simulink model "raibert_controller"  (R2018b)
settings: Solver=FixedStepDiscrete  StartTime=0.0  StopTime=inf  FixedStep=sample_time  RelTol=1e-3
InitFcn:
  | addpath('../common/')
  | simulation_params
  | mechanical_params
values from neighbouring files (symbols this model uses):
  sample_time = 1/sample_freq    (= 0.001)    [simulation_params.m]
undefined symbols (not defined in the file or in its folder): F_thrust, Force_Control, K_d_hip, K_p_hip, K_v, sm, v_avg
libraries: powerlib_meascontrol x1
settings Model: Creator=wmartin  LastModifiedBy=akhadke
settings DataIOCC: SaveFormat=StructureWithTime  SaveOutput=off  SignalLogging=off  DSMLogging=off  SaveTime=off
settings OptimizationCC: BlockReduction=off  DefaultParameterBehavior=Inlined  UseFloatMulNetSlope=on  InlineInvariantSignals=on  OptimizeBlockIOStorage=off  BufferReuse=off  GlobalBufferReuse=off  ExpressionFolding=off  LocalBlockOutputs=off  LifeSpan=0.5  SimCompilerOptimization=on  OptimizeDataStoreBuffers=off  BusAssignmentInplaceUpdate=off
settings DebuggingCC: UnderspecifiedInitializationDetection=Classic  MergeDetectMultiDrivingBlocksExec=none  LibraryContextMissingDiagnostic=none
settings HardwareCC: ProdBitPerPointer=32  ProdBitPerSizeT=32  ProdBitPerPtrDiffT=32  ProdLargestAtomicFloat=None  ProdWordSize=32  ProdLongLongMode=on  ProdHWDeviceType=Generic->32-bit x86 compatible
settings ModelReferenceCC: ModelReferenceNumInstancesAllowed=Single  ModelReferenceMinAlgLoopOccurrences=on  PropagateSignalLabelsOutOfModel=off
settings SFSimCC: SimUseLocalCustomCode=off
settings RTWCC: SystemTargetFile=slrt.tlc  TLCOptions=-axPCModelStackSizeKB=1024  TemplateMakefile=slrt_default_tmf  Description=Simulink Real-Time  RTWUseLocalCustomCode=off  CodeExecutionProfiling=on  RTWCompilerOptimization=on
settings CodeAppCC: MaxIdLength=127  StateflowObjectComments=on
settings TargetCC: CodeReplacementLibrary=XPC_BLAS  ParMdlRefBuildCompliant=on  ConcurrentExecutionCompliant=on  GeneratePreprocessorConditionals=Use local settings  MatFileLogging=on  PreserveStateflowLocalDataDimensions=off  MATLABClassNameForMDSCustomization=xpcAperiodicCustomization

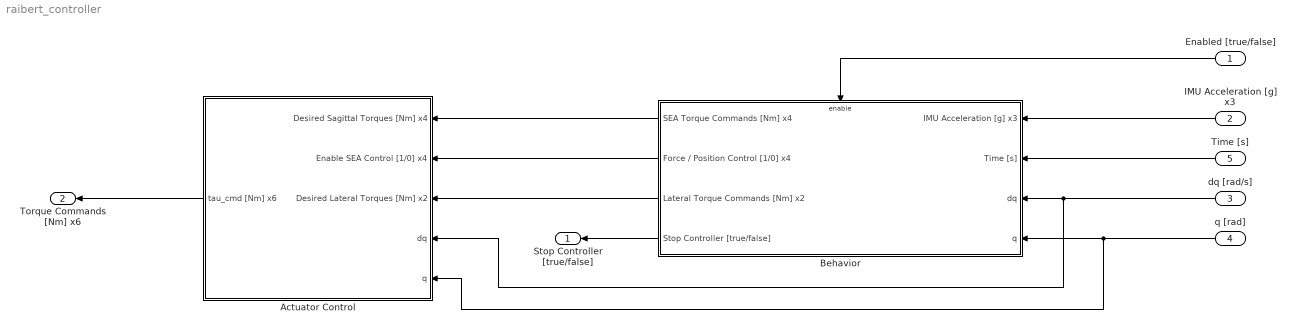
== system raibert_controller ==
  Enabled [true/false] : Inport  OutDataTypeStr=boolean  PortDimensions=1  SampleTime=sample_time  Interpolate=off
  IMU Acceleration [g] x3 : Inport  Port=2  OutDataTypeStr=double  PortDimensions=3  SampleTime=[0.001,0]  Interpolate=off
  dq [rad/s] : Inport  Port=3  OutDataTypeStr=double  PortDimensions=13  SampleTime=[0.001,0]  Interpolate=off
  q [rad] : Inport  Port=4  OutDataTypeStr=double  PortDimensions=13  SampleTime=[0.001,0]  Interpolate=off
  Time [s] : Inport  Port=5  OutDataTypeStr=double  PortDimensions=1  SampleTime=sample_time  Interpolate=off
  Actuator Control : Subsystem
  Behavior : Subsystem
  Stop Controller [true/false] : Outport  OutDataTypeStr=boolean  PortDimensions=1  SampleTime=[0.001,0]  OutputWhenDisabled=reset  InitialOutput=[0 0 0 0 0 0]
  Torque Commands [Nm] x6 : Outport  Port=2  OutDataTypeStr=double  PortDimensions=6  SampleTime=[0.001,0]  OutputWhenDisabled=reset  InitialOutput=[0 0 0 0 0 0]
  wires:
  IMU Acceleration [g] x3/1 -> Behavior/1(IMU Acceleration [g] x3)
  dq [rad/s]/1 -> Behavior/3(dq), Actuator Control/4(dq)
  q [rad]/1 -> Behavior/4(q), Actuator Control/5(q)
  Time [s]/1 -> Behavior/2(Time [s])
  Enabled [true/false]/1 -> Behavior/Enable
  Behavior/4(Stop Controller [true/false]) -> Stop Controller [true/false]/1
  Behavior/2(Force / Position Control [1/0] x4) -> Actuator Control/2(Enable SEA Control [1/0] x4)
  Actuator Control/1(tau_cmd [Nm] x6) -> Torque Commands [Nm] x6/1
  Behavior/1(SEA Torque Commands [Nm] x4) -> Actuator Control/1(Desired Sagittal Torques [Nm] x4)
  Behavior/3(Lateral Torque Commands [Nm] x2) -> Actuator Control/3(Desired Lateral Torques [Nm] x2)

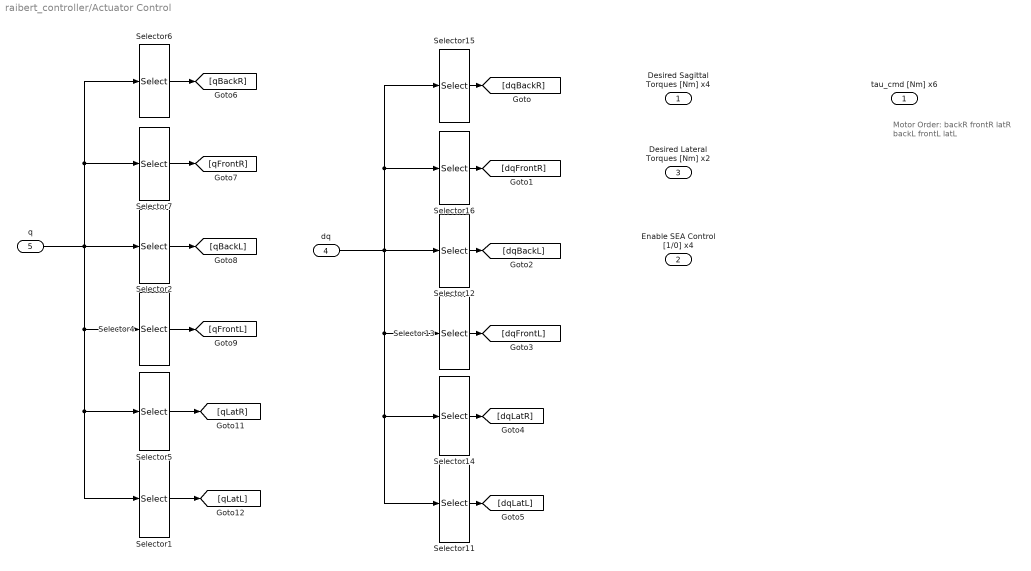
== system raibert_controller/Actuator Control ==
  note: Motor Order:
      |
      | backR
      | frontR
      | latR
      | backL
      | frontL
      | latL
  Desired Sagittal Torques [Nm] x4 : Inport  OutDataTypeStr=double  PortDimensions=4  SampleTime=sample_time
  Enable SEA Control [1/0] x4 : Inport  Port=2  OutDataTypeStr=boolean  PortDimensions=4  SampleTime=sample_time
  Desired Lateral Torques [Nm] x2 : Inport  Port=3  OutDataTypeStr=double  PortDimensions=2  SampleTime=sample_time
  dq : Inport  Port=4  OutDataTypeStr=double  PortDimensions=13  SampleTime=sample_time
  q : Inport  Port=5  OutDataTypeStr=double  PortDimensions=13  SampleTime=sample_time
  Selector1 : Selector  InputPortWidth=13  IndexOptions=Index vector (dialog)  Indices=[10]  OutputSizes=1
  Selector11 : Selector  InputPortWidth=13  IndexOptions=Index vector (dialog)  Indices=[10]  OutputSizes=1
  Selector12 : Selector  InputPortWidth=13  IndexOptions=Index vector (dialog)  Indices=[5 6]  OutputSizes=1
  Selector13 : Selector  InputPortWidth=13  IndexOptions=Index vector (dialog)  Indices=[7 8]  OutputSizes=1
  Selector14 : Selector  InputPortWidth=13  IndexOptions=Index vector (dialog)  Indices=[9]  OutputSizes=1
  Selector15 : Selector  InputPortWidth=13  IndexOptions=Index vector (dialog)  Indices=[1 2]  OutputSizes=1
  Selector16 : Selector  InputPortWidth=13  IndexOptions=Index vector (dialog)  Indices=[3 4]  OutputSizes=1
  Selector2 : Selector  InputPortWidth=13  IndexOptions=Index vector (dialog)  Indices=[5 6]  OutputSizes=1
  Selector4 : Selector  InputPortWidth=13  IndexOptions=Index vector (dialog)  Indices=[7 8]  OutputSizes=1
  Selector5 : Selector  InputPortWidth=13  IndexOptions=Index vector (dialog)  Indices=[9]  OutputSizes=1
  Selector6 : Selector  InputPortWidth=13  IndexOptions=Index vector (dialog)  Indices=[1 2]  OutputSizes=1
  Selector7 : Selector  InputPortWidth=13  IndexOptions=Index vector (dialog)  Indices=[3 4]  OutputSizes=1
  tau_cmd [Nm] x6 : Outport  OutDataTypeStr=double  PortDimensions=6  InitialOutput=[0 0 0 0 0 0]
  wires:
  Selector15/1 -> [dqBackR]
  Selector13/1 -> [dqFrontL]
  Selector1/1 -> [qLatL]
  Selector12/1 -> [dqBackL]
  Selector2/1 -> [qBackL]
  Selector4/1 -> [qFrontL]
  Selector5/1 -> [qLatR]
  Selector6/1 -> [qBackR]
  dq/1 -> Selector12/1, Selector16/1, Selector15/1, Selector13/1, Selector14/1, Selector11/1
  Selector11/1 -> [dqLatL]
  q/1 -> Selector1/1, Selector5/1, Selector4/1, Selector6/1, Selector7/1, Selector2/1
  Selector7/1 -> [qFrontR]
  Selector16/1 -> [dqFrontR]
  Selector14/1 -> [dqLatR]

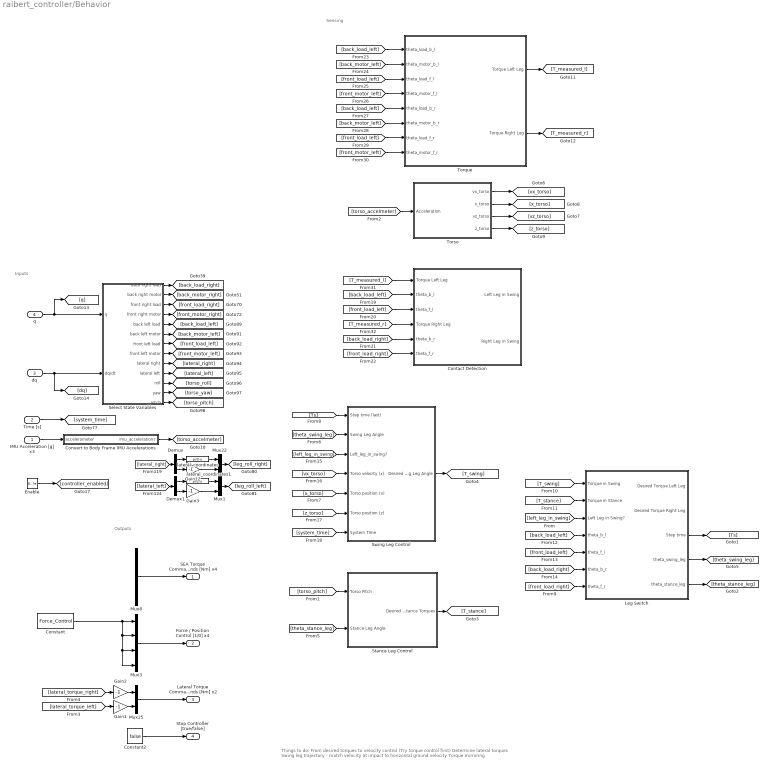
== system raibert_controller/Behavior ==
  note: Things to do:
      | From desired torques to velocity control (Try torque control first)
      | Determine lateral torques
      | Swing leg trajectory - match velocity at impact to horizontal ground velocity
      | Torque mirroring
  note: Outputs
  note: Sensing
  note: Inputs
  IMU Acceleration [g] x3 : Inport  OutDataTypeStr=double  PortDimensions=3  SampleTime=[0.001,0]
  Time [s] : Inport  Port=2  OutDataTypeStr=double  PortDimensions=1  SampleTime=[0.001,0]
  dq : Inport  Port=3  OutDataTypeStr=double  PortDimensions=13  SampleTime=[0.001,0]
  q : Inport  Port=4  OutDataTypeStr=double  PortDimensions=13  SampleTime=[0.001,0]
  Enable : EnablePort  PropagateVarSize=During execution  ShowOutputPort=on
  Constant : Constant  Value=Force_Control
  Constant2 : Constant  Value=false
  Contact Detection : Subsystem
  Convert to Body Frame IMU Accelerations : MATLAB Function  TreatAsAtomicUnit=on
  Demux : Demux  Outputs=2
  Demux1 : Demux  Outputs=2
  Gain{1..3,12} (4 alike) : Gain  Gain=-1
  Leg Switch : Subsystem
  Mux1 : Mux  Inputs=2
  Mux22 : Mux  Inputs=2
  Mux25 : Mux  Inputs=2
  Mux3 : Mux
  Mux8 : Mux
  Select State Variables : Subsystem
  Stance Leg Control : Subsystem  TreatAsAtomicUnit=on
  Swing Leg Control : Subsystem  TreatAsAtomicUnit=on
  Torque : Subsystem
  Torso : Subsystem
  lateral_coordinates : Fcn  Expr=pi/2-u
  lateral_coordinates1 : Fcn  Expr=pi/2-u
  SEA Torque Commands [Nm] x4 : Outport  OutDataTypeStr=double  PortDimensions=4  SampleTime=[0.001,0]  OutputWhenDisabled=reset  InitialOutput=[0 0 0 0]
  Force / Position Control [1/0] x4 : Outport  Port=2  OutDataTypeStr=boolean  PortDimensions=4  SampleTime=[0.001,0]  OutputWhenDisabled=reset  InitialOutput=[0 0 0 0]
  Lateral Torque Commands [Nm] x2 : Outport  Port=3  OutDataTypeStr=double  PortDimensions=2  SampleTime=[0.001,0]  OutputWhenDisabled=reset  InitialOutput=[0 0]
  Stop Controller [true/false] : Outport  Port=4  OutDataTypeStr=boolean  PortDimensions=1  SampleTime=[0.001,0]  OutputWhenDisabled=reset  InitialOutput=0
  wires:
  Time [s]/1 -> [system_time]
  Demux/2 -> Gain12/1
  lateral_coordinates/1 -> Mux22/1
  Gain12/1 -> Mux22/2
  Mux22/1 -> [leg_roll_right]
  Demux/1 -> lateral_coordinates/1
  [lateral_torque_right] -> Gain2/1
  q/1 -> [q], Select State Variables/1(q)
  [lateral_torque_left] -> Gain1/1
  Mux8/1 -> SEA Torque Commands [Nm] x4/1
  Mux3/1 -> Force / Position Control [1/0] x4/1
  Gain2/1 -> Mux25/1
  Mux25/1 -> Lateral Torque Commands [Nm] x2/1
  Gain1/1 -> Mux25/2
  Constant2/1 -> Stop Controller [true/false]/1
  dq/1 -> [dq], Select State Variables/2(dq/dt)
  Select State Variables/1(back right load) -> [back_load_right]
  Select State Variables/2(back right motor) -> [back_motor_right]
  Select State Variables/3(front right load) -> [front_load_right]
  Select State Variables/4(front right motor) -> [front_motor_right]
  Select State Variables/5(back left load) -> [back_load_left]
  Select State Variables/6(back left motor) -> [back_motor_left]
  Select State Variables/7(front left load) -> [front_load_left]
  Select State Variables/8(front left motor) -> [front_motor_left]
  Select State Variables/13(pitch) -> [torso_pitch]
  Select State Variables/12(yaw) -> [torso_yaw]
  Select State Variables/11(roll) -> [torso_roll]
  Select State Variables/10(lateral left) -> [lateral_left]
  Select State Variables/9(lateral right) -> [lateral_right]
  [lateral_right] -> Demux/1
  [lateral_left] -> Demux1/1
  Demux1/1 -> lateral_coordinates1/1
  Mux1/1 -> [leg_roll_left]
  Gain3/1 -> Mux1/2
  lateral_coordinates1/1 -> Mux1/1
  Demux1/2 -> Gain3/1
  Enable/1 -> [controller_enabled]
  Convert to Body Frame IMU Accelerations/1(imu_accelerations) -> [torso_accelmeter]
  IMU Acceleration [g] x3/1 -> Convert to Body Frame IMU Accelerations/1(accelerometer)
  Leg Switch/3(Step time) -> [Ts]
  [torso_pitch] -> Stance Leg Control/1(Torso Pitch)
  [vx_torso] -> Swing Leg Control/4(Torso velocity (x))
  [Ts] -> Swing Leg Control/1(Step time (last))
  [torso_accelmeter] -> Torso/1(Acceleration)
  Stance Leg Control/1(Desired Stance Torques) -> [T_stance]
  Swing Leg Control/1(Desired Swing Leg Angle) -> [T_swing]
  [T_swing] -> Leg Switch/1(Torque in Swing)
  [T_stance] -> Leg Switch/2(Torque in Stance)
  [back_load_right] -> Leg Switch/6(theta_b_r)
  [front_load_right] -> Leg Switch/7(theta_f_r)
  [back_load_left] -> Leg Switch/4(theta_b_l)
  [front_load_left] -> Leg Switch/5(theta_f_l)
  Leg Switch/4(theta_swing_leg) -> [theta_swing_leg]
  [theta_swing_leg] -> Swing Leg Control/2(Swing Leg Angle)
  Constant/1 -> Mux3/4, Mux3/3, Mux3/2, Mux3/1
  [left_leg_in_swing] -> Leg Switch/3("Left Leg in Swing? ")
  [left_leg_in_swing] -> Swing Leg Control/3(Left_leg_in_swing?)
  Torso/1(vx_torso) -> [vx_torso]
  Torso/3(vz_torso) -> [vz_torso]
  Torso/2(x_torso) -> [x_torso]
  Torso/4(z_torso) -> [z_torso]
  [x_torso] -> Swing Leg Control/5(Torso position (x))
  [z_torso] -> Swing Leg Control/6(Torso position (z))
  [system_time] -> Swing Leg Control/7(System Time)
  Leg Switch/5(theta_stance_leg) -> [theta_stance_leg]
  [theta_stance_leg] -> Stance Leg Control/2(Stance Leg Angle)
  [back_load_left] -> Contact Detection/2(theta_b_l)
  [front_load_left] -> Contact Detection/3(theta_f_l)
  [back_load_right] -> Contact Detection/5(theta_b_r)
  [front_load_right] -> Contact Detection/6(theta_f_r)
  [back_load_left] -> Torque/1(theta_load_b_l)
  [back_motor_left] -> Torque/2(theta_motor_b_l)
  [front_load_left] -> Torque/3(theta_load_f_l)
  [front_motor_left] -> Torque/4(theta_motor_f_l)
  [back_load_left] -> Torque/5(theta_load_b_r)
  [back_motor_left] -> Torque/6(theta_motor_b_r)
  [front_load_left] -> Torque/7(theta_load_f_r)
  [front_motor_left] -> Torque/8(theta_motor_f_r)
  Torque/1(Torque Left Leg) -> [T_measured_l]
  Torque/2(Torque Right Leg) -> [T_measured_r]
  [T_measured_l] -> Contact Detection/1(Torque Left Leg)
  [T_measured_r] -> Contact Detection/4(Torque Right Leg)

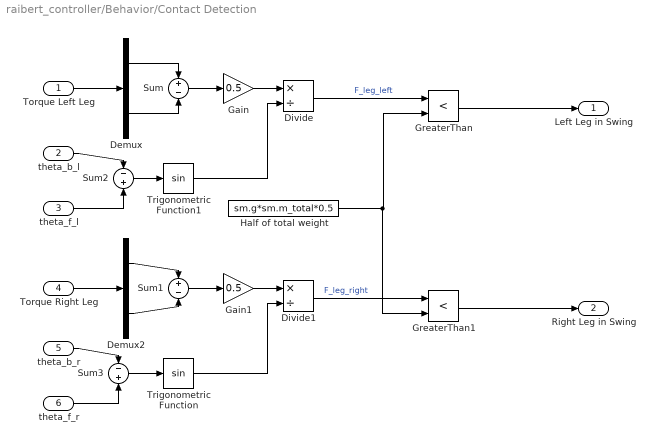
== system raibert_controller/Behavior/Contact Detection ==
  Torque Left Leg : Inport
  theta_b_l : Inport  Port=2
  theta_f_l : Inport  Port=3
  Torque Right Leg : Inport  Port=4
  theta_b_r : Inport  Port=5
  theta_f_r : Inport  Port=6
  Demux : Demux  Outputs=2
  Demux2 : Demux  Outputs=2
  Divide : Product  Inputs=*/
  Divide1 : Product  Inputs=*/
  Gain : Gain  Gain=0.5
  Gain1 : Gain  Gain=0.5
  GreaterThan : RelationalOperator  Operator=<  OutDataTypeStr=boolean  RndMeth=Simplest
  GreaterThan1 : RelationalOperator  Operator=<  OutDataTypeStr=boolean  RndMeth=Simplest
  Half of total weight : Constant  Value=sm.g*sm.m_total*0.5
  Sum : Sum  Inputs=+-
  Sum1 : Sum  Inputs=+-
  Sum2 : Sum  Inputs=-+
  Sum3 : Sum  Inputs=-+
  Trigonometric Function : Trigonometry
  Trigonometric Function1 : Trigonometry
  Left Leg in Swing : Outport
  Right Leg in Swing : Outport  Port=2
  wires:
  Torque Left Leg/1 -> Demux/1
  Demux/1 -> Sum/1
  Demux/2 -> Sum/2
  Torque Right Leg/1 -> Demux2/1
  Demux2/1 -> Sum1/1
  Demux2/2 -> Sum1/2
  Sum/1 -> Gain/1
  Sum1/1 -> Gain1/1
  theta_f_l/1 -> Sum2/2
  theta_b_l/1 -> Sum2/1
  theta_f_r/1 -> Sum3/2
  theta_b_r/1 -> Sum3/1
  Sum3/1 -> Trigonometric Function/1
  Sum2/1 -> Trigonometric Function1/1
  Gain/1 -> Divide/1
  Trigonometric Function1/1 -> Divide/2
  Gain1/1 -> Divide1/1
  Trigonometric Function/1 -> Divide1/2
  Divide/1 -> GreaterThan/1  "F_leg_left"
  Divide1/1 -> GreaterThan1/1  "F_leg_right"
  Half of total weight/1 -> GreaterThan1/2, GreaterThan/2
  GreaterThan/1 -> Left Leg in Swing/1
  GreaterThan1/1 -> Right Leg in Swing/1

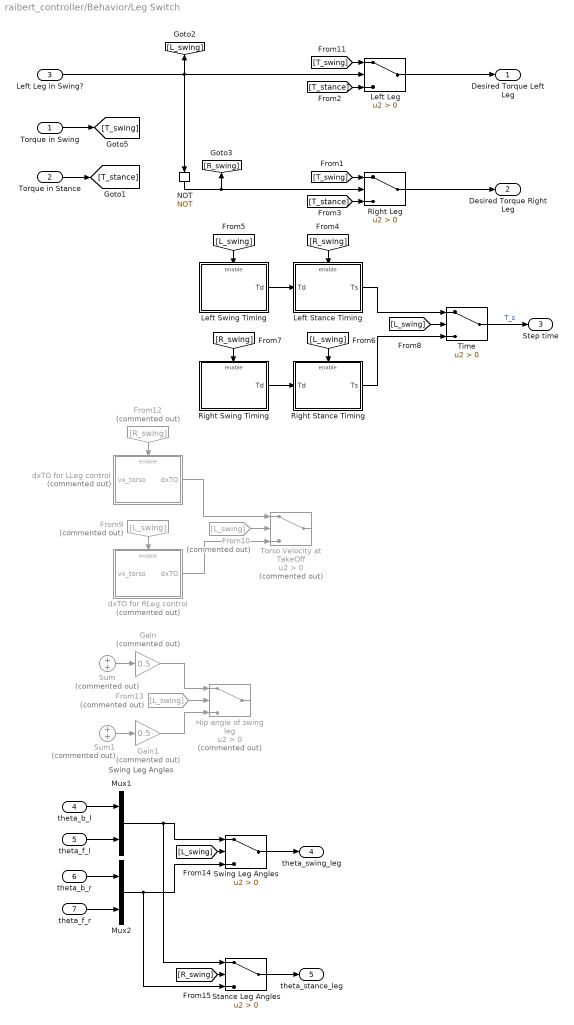
== system raibert_controller/Behavior/Leg Switch ==
  note: Swing Leg Angles
  Torque in Swing : Inport
  Torque in Stance : Inport  Port=2
  "Left Leg in Swing? " : Inport  Port=3
  theta_b_l : Inport  Port=4
  theta_f_l : Inport  Port=5
  theta_b_r : Inport  Port=6
  theta_f_r : Inport  Port=7
  From10 : From  Commented=on  GotoTag=L_swing
  From12 : From  Commented=on  GotoTag=R_swing
  From13 : From  Commented=on  GotoTag=L_swing
  From9 : From  Commented=on  GotoTag=L_swing
  Gain : Gain  Commented=on  Gain=0.5
  Gain1 : Gain  Commented=on  Gain=0.5
  Hip angle of swing leg : Switch  Commented=on  Criteria=u2 > Threshold
  Left Leg : Switch  Criteria=u2 > Threshold
  Left Stance Timing : Subsystem
  Left Swing Timing : Subsystem
  Mux1 : Mux  Inputs=2
  Mux2 : Mux  Inputs=2
  NOT : Logic  Operator=NOT  IconShape=distinctive  AllPortsSameDT=off  OutDataTypeStr=boolean
  Right Leg : Switch  Criteria=u2 > Threshold
  Right Stance Timing : Subsystem
  Right Swing Timing : Subsystem
  Stance Leg Angles : Switch  Criteria=u2 > Threshold
  Sum : Sum  Commented=on
  Sum1 : Sum  Commented=on
  Swing Leg Angles : Switch  Criteria=u2 > Threshold
  Time : Switch  Criteria=u2 > Threshold
  Torso Velocity at TakeOff : Switch  Commented=on  Criteria=u2 > Threshold
  dxTO for LLeg control : Subsystem  Commented=on
  dxTO for RLeg control : Subsystem  Commented=on
  Desired Torque Left Leg : Outport
  Desired Torque Right Leg : Outport  Port=2
  Step time : Outport  Port=3
  theta_swing_leg : Outport  Port=4
  theta_stance_leg : Outport  Port=5
  wires:
  "Left Leg in Swing? "/1 -> NOT/1, Left Leg/2, [L_swing]
  NOT/1 -> [R_swing], Right Leg/2
  Torque in Swing/1 -> [T_swing]
  Torque in Stance/1 -> [T_stance]
  [T_swing] -> Left Leg/1
  [T_swing] -> Right Leg/1
  [T_stance] -> Left Leg/3
  [T_stance] -> Right Leg/3
  Left Leg/1 -> Desired Torque Left Leg/1
  Left Swing Timing/1(Td) -> Left Stance Timing/1(Td)
  Right Swing Timing/1(Td) -> Right Stance Timing/1(Td)
  [L_swing] -> Left Swing Timing/Enable
  [L_swing] -> Right Stance Timing/Enable
  [R_swing] -> Left Stance Timing/Enable
  [R_swing] -> Right Swing Timing/Enable
  Time/1 -> Step time/1  "T_s"
  Left Stance Timing/1(Ts) -> Time/1
  Right Stance Timing/1(Ts) -> Time/3
  [L_swing] -> Time/2
  From9/1 -> dxTO for RLeg control/Enable
  From12/1 -> dxTO for LLeg control/Enable
  dxTO for LLeg control/1(dxTO) -> Torso Velocity at TakeOff/1
  From10/1 -> Torso Velocity at TakeOff/2
  dxTO for RLeg control/1(dxTO) -> Torso Velocity at TakeOff/3
  Sum/1 -> Gain/1
  Sum1/1 -> Gain1/1
  From13/1 -> Hip angle of swing leg/2
  Gain/1 -> Hip angle of swing leg/1
  Gain1/1 -> Hip angle of swing leg/3
  theta_b_l/1 -> Mux1/1
  theta_f_l/1 -> Mux1/2
  theta_b_r/1 -> Mux2/1
  theta_f_r/1 -> Mux2/2
  [L_swing] -> Swing Leg Angles/2
  Swing Leg Angles/1 -> theta_swing_leg/1
  Stance Leg Angles/1 -> theta_stance_leg/1
  Mux2/1 -> Stance Leg Angles/3, Swing Leg Angles/3
  Mux1/1 -> Stance Leg Angles/1, Swing Leg Angles/1
  [R_swing] -> Stance Leg Angles/2
  Right Leg/1 -> Desired Torque Right Leg/1

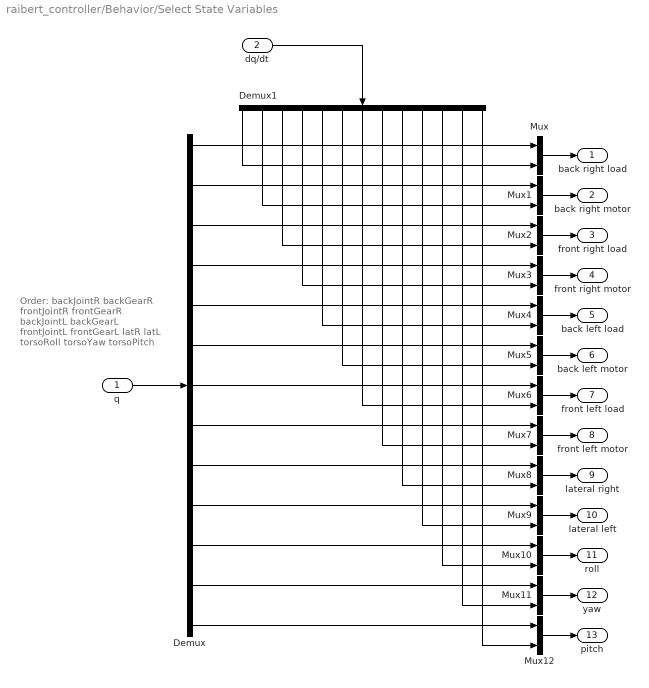
== system raibert_controller/Behavior/Select State Variables ==
  note: Order:
      |
      | backJointR
      | backGearR
      | frontJointR
      | frontGearR
      |
      | backJointL
      | backGearL
      | frontJointL
      | frontGearL
      |
      | latR
      | latL
      |
      | torsoRoll
      | torsoYaw
      | torsoPitch
  q : Inport
  dq/dt : Inport  Port=2
  Demux : Demux  Outputs=13
  Demux1 : Demux  Outputs=13
  Mux{,1..12} (13 alike) : Mux  Inputs=2
  back right load : Outport
  back right motor : Outport  Port=2
  front right load : Outport  Port=3
  front right motor : Outport  Port=4
  back left load : Outport  Port=5
  back left motor : Outport  Port=6
  front left load : Outport  Port=7
  front left motor : Outport  Port=8
  lateral right : Outport  Port=9
  lateral left : Outport  Port=10
  roll : Outport  Port=11
  yaw : Outport  Port=12
  pitch : Outport  Port=13
  wires:
  q/1 -> Demux/1
  dq/dt/1 -> Demux1/1
  Mux/1 -> back right load/1
  Mux1/1 -> back right motor/1
  Mux4/1 -> back left load/1
  Mux5/1 -> back left motor/1
  Mux8/1 -> lateral right/1
  Mux9/1 -> lateral left/1
  Mux12/1 -> pitch/1
  Mux2/1 -> front right load/1
  Mux3/1 -> front right motor/1
  Mux6/1 -> front left load/1
  Mux7/1 -> front left motor/1
  Mux10/1 -> roll/1
  Mux11/1 -> yaw/1
  Demux/1 -> Mux/1
  Demux1/1 -> Mux/2
  Demux/2 -> Mux1/1
  Demux/3 -> Mux2/1
  Demux/4 -> Mux3/1
  Demux/5 -> Mux4/1
  Demux/6 -> Mux5/1
  Demux/7 -> Mux6/1
  Demux/8 -> Mux7/1
  Demux/9 -> Mux8/1
  Demux/10 -> Mux9/1
  Demux/11 -> Mux10/1
  Demux/12 -> Mux11/1
  Demux/13 -> Mux12/1
  Demux1/2 -> Mux1/2
  Demux1/3 -> Mux2/2
  Demux1/4 -> Mux3/2
  Demux1/5 -> Mux4/2
  Demux1/6 -> Mux5/2
  Demux1/7 -> Mux6/2
  Demux1/8 -> Mux7/2
  Demux1/9 -> Mux8/2
  Demux1/10 -> Mux9/2
  Demux1/11 -> Mux10/2
  Demux1/12 -> Mux11/2
  Demux1/13 -> Mux12/2

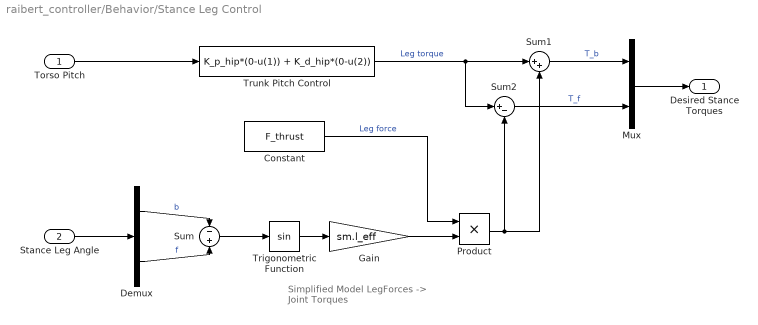
== system raibert_controller/Behavior/Stance Leg Control ==
  note: Simplified Model
      | LegForces -> Joint Torques
  Torso Pitch : Inport
  Stance Leg Angle : Inport  Port=2
  Constant : Constant  Value=F_thrust
  Demux : Demux  Outputs=2
  Gain : Gain  Gain=sm.l_eff
  Mux : Mux  Inputs=2
  Product : Product
  Sum : Sum  Inputs=-+
  Sum1 : Sum  Inputs=|++
  Sum2 : Sum  Inputs=|+-
  Trigonometric Function : Trigonometry
  Trunk Pitch Control : Fcn  Expr=K_p_hip*(0-u(1)) + K_d_hip*(0-u(2))
  Desired Stance Torques : Outport  OutputWhenDisabled=reset  InitialOutput=0
  wires:
  Torso Pitch/1 -> Trunk Pitch Control/1
  Trunk Pitch Control/1 -> Sum2/1, Sum1/1  "Leg torque"
  Mux/1 -> Desired Stance Torques/1
  Constant/1 -> Product/1  "Leg force"
  Stance Leg Angle/1 -> Demux/1
  Demux/1 -> Sum/1  "b"
  Demux/2 -> Sum/2  "f"
  Sum/1 -> Trigonometric Function/1
  Trigonometric Function/1 -> Gain/1
  Gain/1 -> Product/2
  Product/1 -> Sum1/2, Sum2/2
  Sum2/1 -> Mux/2  "T_f"
  Sum1/1 -> Mux/1  "T_b"

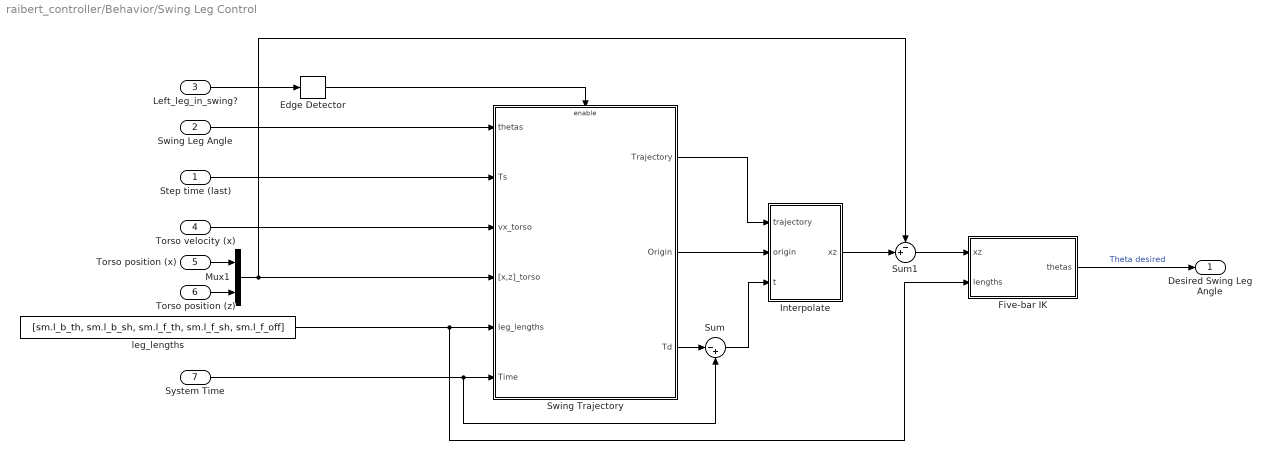
== system raibert_controller/Behavior/Swing Leg Control ==
  Step time (last) : Inport
  Swing Leg Angle : Inport  Port=2
  Left_leg_in_swing? : Inport  Port=3
  Torso velocity (x) : Inport  Port=4
  Torso position (x) : Inport  Port=5
  Torso position (z) : Inport  Port=6
  System Time : Inport  Port=7
  Edge Detector : powerlib_meascontrol/Logic/Edge Detector  model=Either  ic=0  Ts=0
      settings: SourceProductName=Simscape Power Systems  SourceProductBaseCode=PS
  Five-bar IK : MATLAB Function  TreatAsAtomicUnit=on
  Interpolate : MATLAB Function  TreatAsAtomicUnit=on
  Mux1 : Mux  Inputs=2
  Sum : Sum  Inputs=|-+
  Sum1 : Sum  Inputs=-+|
  Swing Trajectory : Subsystem
  leg_lengths : Constant  Value=[sm.l_b_th, sm.l_b_sh, sm.l_f_th, sm.l_f_sh, sm.l_f_off]
  Desired Swing Leg Angle : Outport  OutputWhenDisabled=reset  InitialOutput=0
  wires:
  Edge Detector/1 -> Swing Trajectory/Enable
  Left_leg_in_swing?/1 -> Edge Detector/1
  Step time (last)/1 -> Swing Trajectory/2(Ts)
  Torso velocity (x)/1 -> Swing Trajectory/3(vx_torso)
  Torso position (x)/1 -> Mux1/1
  Torso position (z)/1 -> Mux1/2
  Mux1/1 -> Sum1/1, Swing Trajectory/4("[x,z]_torso")
  Swing Leg Angle/1 -> Swing Trajectory/1(thetas)
  System Time/1 -> Swing Trajectory/6(Time), Sum/2
  Swing Trajectory/1(Trajectory) -> Interpolate/1(trajectory)
  Swing Trajectory/3(Td) -> Sum/1
  Sum/1 -> Interpolate/3(t)
  Swing Trajectory/2(Origin) -> Interpolate/2(origin)
  leg_lengths/1 -> Five-bar IK/2(lengths), Swing Trajectory/5(leg_lengths)
  Interpolate/1(xz) -> Sum1/2
  Sum1/1 -> Five-bar IK/1(xz)
  Five-bar IK/1(thetas) -> Desired Swing Leg Angle/1  "Theta desired"

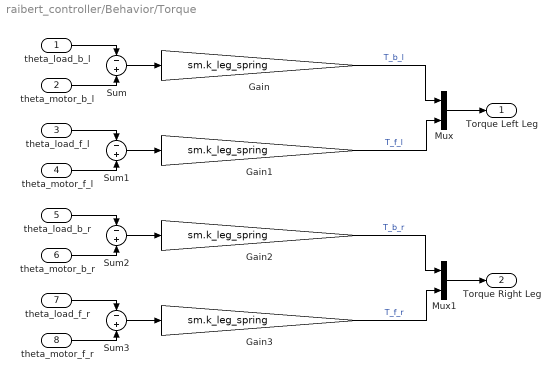
== system raibert_controller/Behavior/Torque ==
  theta_load_b_l : Inport
  theta_motor_b_l : Inport  Port=2
  theta_load_f_l : Inport  Port=3
  theta_motor_f_l : Inport  Port=4
  theta_load_b_r : Inport  Port=5
  theta_motor_b_r : Inport  Port=6
  theta_load_f_r : Inport  Port=7
  theta_motor_f_r : Inport  Port=8
  Gain{,1..3} (4 alike) : Gain  Gain=sm.k_leg_spring
  Mux : Mux  Inputs=2
  Mux1 : Mux  Inputs=2
  Sum{,1..3} (4 alike) : Sum  Inputs=-+
  Torque Left Leg : Outport
  Torque Right Leg : Outport  Port=2
  wires:
  theta_motor_b_l/1 -> Sum/2
  theta_load_b_l/1 -> Sum/1
  Sum/1 -> Gain/1
  Gain/1 -> Mux/1  "T_b_l"
  Gain1/1 -> Mux/2  "T_f_l"
  theta_motor_f_l/1 -> Sum1/2
  theta_load_f_l/1 -> Sum1/1
  Sum1/1 -> Gain1/1
  Mux/1 -> Torque Left Leg/1
  theta_load_b_r/1 -> Sum2/1
  Sum2/1 -> Gain2/1
  Gain3/1 -> Mux1/2  "T_f_r"
  theta_motor_b_r/1 -> Sum2/2
  Mux1/1 -> Torque Right Leg/1
  Gain2/1 -> Mux1/1  "T_b_r"
  Sum3/1 -> Gain3/1
  theta_load_f_r/1 -> Sum3/1
  theta_motor_f_r/1 -> Sum3/2

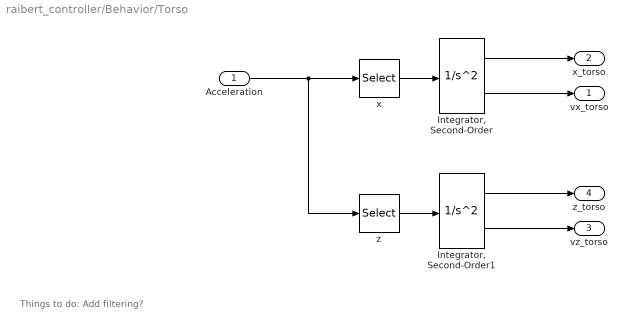
== system raibert_controller/Behavior/Torso ==
  note: Things to do:
      | Add filtering?
  Acceleration : Inport
  "Integrator, Second-Order" : SecondOrderIntegrator  ICX=0
  "Integrator, Second-Order1" : SecondOrderIntegrator  ICX=sm.initial_com_height
  x : Selector  InputPortWidth=3  IndexOptions=Index vector (dialog)  Indices=[1]  OutputSizes=1
  z : Selector  InputPortWidth=3  IndexOptions=Index vector (dialog)  Indices=[3]  OutputSizes=1
  vx_torso : Outport
  x_torso : Outport  Port=2
  vz_torso : Outport  Port=3
  z_torso : Outport  Port=4
  wires:
  Acceleration/1 -> z/1, x/1
  x/1 -> "Integrator, Second-Order"/1
  z/1 -> "Integrator, Second-Order1"/1
  "Integrator, Second-Order1"/2 -> vz_torso/1
  "Integrator, Second-Order"/2 -> vx_torso/1
  "Integrator, Second-Order"/1 -> x_torso/1
  "Integrator, Second-Order1"/1 -> z_torso/1

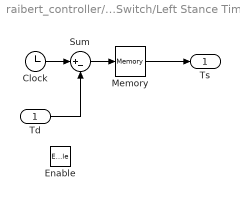
== system raibert_controller/Behavior/Leg Switch/Left Stance Timing ==
  Td : Inport
  Enable : EnablePort
  Clock : Clock
  Memory : Memory
  Sum : Sum  Inputs=|+-
  Ts : Outport
  wires:
  Clock/1 -> Sum/1
  Td/1 -> Sum/2
  Memory/1 -> Ts/1
  Sum/1 -> Memory/1

== system raibert_controller/Behavior/Leg Switch/Left Swing Timing ==
  Enable : EnablePort
  Clock : Clock
  Td : Outport
  wires:
  Clock/1 -> Td/1

== system raibert_controller/Behavior/Leg Switch/Right Stance Timing ==
  Td : Inport
  Enable : EnablePort
  Clock : Clock
  Memory : Memory
  Sum : Sum  Inputs=|+-
  Ts : Outport
  wires:
  Clock/1 -> Sum/1
  Td/1 -> Sum/2
  Memory/1 -> Ts/1
  Sum/1 -> Memory/1

== system raibert_controller/Behavior/Leg Switch/Right Swing Timing ==
  Enable : EnablePort
  Clock : Clock
  Td : Outport
  wires:
  Clock/1 -> Td/1

== system raibert_controller/Behavior/Leg Switch/dxTO for LLeg control ==
  vx_torso : Inport
  Enable : EnablePort
  dxTO : Outport
  wires:
  vx_torso/1 -> dxTO/1

== system raibert_controller/Behavior/Leg Switch/dxTO for RLeg control ==
  vx_torso : Inport
  Enable : EnablePort
  dxTO : Outport
  wires:
  vx_torso/1 -> dxTO/1

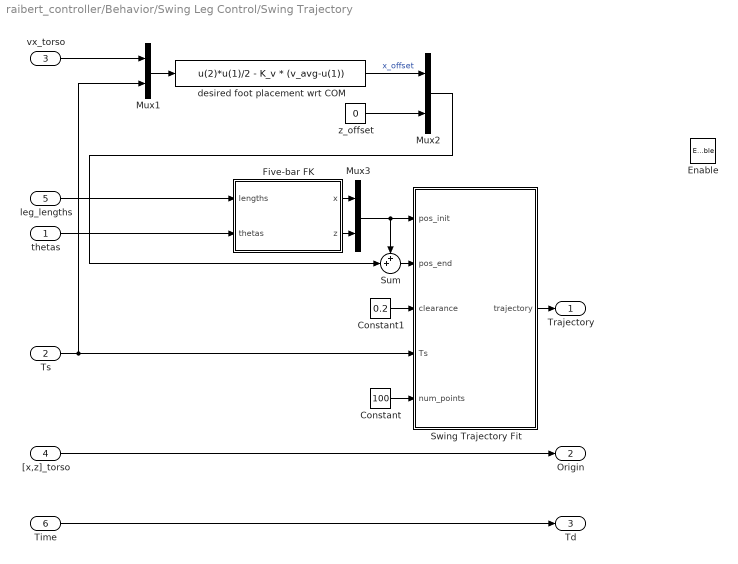
== system raibert_controller/Behavior/Swing Leg Control/Swing Trajectory ==
  thetas : Inport
  Ts : Inport  Port=2
  vx_torso : Inport  Port=3
  "[x,z]_torso" : Inport  Port=4
  leg_lengths : Inport  Port=5
  Time : Inport  Port=6
  Enable : EnablePort
  Constant : Constant  Value=100
  Constant1 : Constant  Value=0.2
  Five-bar FK : MATLAB Function  TreatAsAtomicUnit=on
  Mux1 : Mux  Inputs=2
  Mux2 : Mux  Inputs=2
  Mux3 : Mux  Inputs=2
  Sum : Sum  Inputs=++|
  Swing Trajectory Fit : MATLAB Function  TreatAsAtomicUnit=on
  desired foot placement wrt COM : Fcn  Expr=u(2)*u(1)/2 - K_v * (v_avg-u(1))
  z_offset : Constant  Value=0
  Trajectory : Outport
  Origin : Outport  Port=2
  Td : Outport  Port=3
  wires:
  Swing Trajectory Fit/1(trajectory) -> Trajectory/1
  Ts/1 -> Mux1/2, Swing Trajectory Fit/4(Ts)
  Mux2/1 -> Sum/2
  Constant/1 -> Swing Trajectory Fit/5(num_points)
  Constant1/1 -> Swing Trajectory Fit/3(clearance)
  Sum/1 -> Swing Trajectory Fit/2(pos_end)
  Mux1/1 -> desired foot placement wrt COM/1
  vx_torso/1 -> Mux1/1
  desired foot placement wrt COM/1 -> Mux2/1  "x_offset"
  z_offset/1 -> Mux2/2
  "[x,z]_torso"/1 -> Origin/1
  thetas/1 -> Five-bar FK/2(thetas)
  Five-bar FK/1(x) -> Mux3/1
  Five-bar FK/2(z) -> Mux3/2
  Mux3/1 -> Swing Trajectory Fit/1(pos_init), Sum/1
  leg_lengths/1 -> Five-bar FK/1(lengths)
  Time/1 -> Td/1

== matlab function raibert_controller/Behavior/Swing Leg Control/Swing Trajectory/Five-bar FK ==
  data: x output; lengths input; z output; thetas input
function [x,z] = fcn(lengths, thetas)
    % theta - [theta_b, theta_f]
    % lengths - [l_b_th, l_b_sh, l_f_th, l_f_sh, l_f_off]
    l1 = lengths(1); % l_b_th
    l2 = lengths(2); % l_b_sh
    l3 = lengths(3); % l_f_th
    l4 = lengths(4); % l_f_sh
    l5 = lengths(5); % l_f_off
    
    assert(thetas(2) > thetas(1), 'Front angle < Back angle');
    
    x_knee_b = l1*cos(thetas(1));
    z_knee_b = l1*sin(thetas(1));
    
    x_knee_f = l3*cos(thetas(2));
    z_knee_f = l3*sin(thetas(2));
    
    theta_hip = thetas(2) - thetas(1);
    theta_ankle = acos((l2^2 + l4^2 - ((x_knee_b-x_knee_f)^2 + (z_knee_b-z_knee_f)^2))/(2*l2*l4));
    
    % 2pi - theta_hip - theta_ankle = theta_knee_f + theta_knee_b
    % l_f_th^2 + l_f_sh^2 - 2(l_f_th)(l_f_sh)cos(theta_knee_f) = l_b_th^2 + l_b_sh^2 - 2(l_b_th)(l_b_sh)cos(theta_knee_b)
    c = 2*pi -theta_hip - theta_ankle;
    alpha = atan2(-l3*l4*sin(c),l1*l2-l3*l4*cos(c));
    if (alpha<0)
        alpha = 2*pi+alpha;
    end
    
    theta_1 = acos((l3^2 + l4^2 - l1^2 - l2^2)/(2*sqrt((l3*l4*sin(c))^2+(l1*l2-l3*l4*cos(c))^2)));
    theta_knee_f1 = alpha + theta_1;
    theta_knee_f2 = alpha - theta_1;
    
    if (theta_knee_f1 > 2*pi)
        theta_knee_f1 = theta_knee_f1 - 2*pi;
    end

    if (theta_knee_f2 < 0)
        theta_knee_f2 = theta_knee_f2 + 2*pi;
    end
    
    if ((theta_knee_f1 > 0) && ((c - theta_knee_f1) > 0))
        theta_knee_f = theta_knee_f1+pi;
    elseif((theta_knee_f2 > 0) && ((c - theta_knee_f2) > 0))
        theta_knee_f = theta_knee_f2+pi;
    end
    
   x = x_knee_f + (l4+l5)*cos(theta_knee_f + thetas(2));
   z = z_knee_f + (l4+l5)*sin(theta_knee_f + thetas(2));
    
end

== matlab function raibert_controller/Behavior/Swing Leg Control/Swing Trajectory/Swing Trajectory Fit ==
  data: pos_init input; trajectory output; pos_end input; clearance input; Ts input; num_points input
function trajectory = fcn(pos_init, pos_end, clearance, Ts, num_points)

    t_points = [0,Ts/2,Ts];
    x_points = [pos_init(1), (pos_init(1) + pos_end(1))/2, pos_end(1)];
    z_points = [pos_init(2), clearance+(pos_init(2) + pos_end(2))/2, pos_end(2)];

    t_q = linspace(0,Ts,num_points);
    x_spline = spline(t_points, x_points, t_q);
    z_spline = spline(t_points, z_points, t_q);
    trajectory = [t_q', x_spline', z_spline'];
    
%     l_th_f = 0.5;
%     l_th_b = 0.5;
%     l_sh_f = 0.4;
%     l_sh_b = 0.4;
%     l_sh_off = 0.15;
%     for i=1:1:size(traj,1)
%         x = traj(i,1);
%         y = traj(i,2);
%         theta_th_f = acos(x/sqrt(x^2+y^2)) - acos((x^2 + y^2 + l_th_f^2 - (l_sh_f+l_sh_off)^2)/((2*l_th_f)*(sqrt(x^2+y^2))));
%     end
    
end

== matlab function raibert_controller/Behavior/Swing Leg Control/Five-bar IK ==
  data: xz input; thetas output; lengths input
function thetas = fcn(xz,lengths)
    % thetas - [theta_b, theta_f] in range [0,2*pi]
    % lengths - [l_b_th, l_b_sh, l_f_th, l_f_sh, l_f_off]
    l1 = lengths(1); % l_b_th
    l2 = lengths(2); % l_b_sh
    l3 = lengths(3); % l_f_th
    l4 = lengths(4); % l_f_sh
    l5 = lengths(5); % l_f_off
    
    x = xz(1);
    z = xz(2);
    thetas = [0,0];
    theta_foot = atan2(z,x);
    if (theta_foot < 0)
        theta_foot = theta_foot + 2*pi;
    end
    d_foot = sqrt(x^2+z^2);
    thetas(2) = theta_foot + acos((d_foot^2 + l3^2 - (l4+l5)^2)/(2*d_foot*l3));
    
    theta_knee_f = pi + acos((l3^2 + (l4+l5)^2 - (x^2+z^2))/(2*l3*(l4+l5)));
    x_ankle = x - l5*cos(theta_knee_f + thetas(2));
    z_ankle = z - l5*sin(theta_knee_f + thetas(2));
    theta_ankle = atan2(z_ankle,x_ankle);
    if (theta_ankle < 0)
        theta_ankle = theta_ankle + 2*pi;
    end
    d_ankle = sqrt(x_ankle^2+z_ankle^2);
    thetas(1) = theta_ankle - acos((d_ankle^2 + l1^2 - l2^2)/(2*d_ankle*l1));
end

== matlab function raibert_controller/Behavior/Swing Leg Control/Interpolate ==
  data: trajectory input; origin input; xz output; t input
function xz = fcn(trajectory, origin, t)
    if (t>trajectory(end,1))
        xz = trajectory(end,2:3);
    else
        xz = zeros(1,2);
        xz(1) = interp1(trajectory(:,1), trajectory(:,2), t);
        xz(2) = interp1(trajectory(:,1), trajectory(:,3), t);
    end
    xz(1) = xz(1) + origin(1);
    xz(2) = xz(2) + origin(2);
end

== matlab function raibert_controller/Behavior/Convert to Body Frame IMU Accelerations ==
  data: accelerometer input; imu_accelerations output
function imu_accelerations = imu_to_body_frame(accelerometer)
    g = 9.803;
    z_up_rotation = [1, 0, 0; 0, 0, 1; 0, -1, 0];
    align_xy_rotation = [sqrt(2)/2, -sqrt(2)/2, 0; sqrt(2)/2, sqrt(2)/2, 0; 0, 0, 1];
    imu_accelerations = g*z_up_rotation*align_xy_rotation*accelerometer;
end
